simulink model "P2_SIL_Model_Diag"  (R2016a)
settings: Solver=ode2  StartTime=0.0  StopTime=Cycle_End  RelTol=1e-3
undefined symbols (not defined in the file): air, APP1_OOR, APP2_OOR, APP_Conversion_IN, APP_Mismatch, bms_inletair_temp, bms_maxchargecurrent, bms_maxdischargecurrent, BMS_Notfallkuehlung, BPP_Flt, cal, clt, ClutchEngag, CrankRequest, dcdc, eng, Engine, EngOverTemp, ENGTRQ_MSMCH_Degraded_CP, ENGTRQ_MSMCH_ErrCritical_CP, ENGTRQ_MSMCH_LimpHome_CP, EngTrqMismatch, env, ess, ESS, ESSOverTemp, fd, FFD, g, gb, Grade, IMG, KeyPos_Flt, KeyPosition, lib_APP_Conversion_IN, lib_ESS_plant_V1_2, lib_OBC_Manager, LossCAN, max_vehicle_rad_air_flow, MCUOverTemp, mot, MotDirMismatch, MotOverTemp, MotTrqMismatch, mph2kph, mph2ms, NeutralGear, obc, OBC_Manager, ParkGear, PRNDL_Flt, ReverseGear, RFD, rho, ShiftLeverPosition, sigbuilder_block, Speed, t_amb, time, tloop ... (+2)
libraries: simulink x104, EC2_libraries x12, Diagnostic x11, lib_CANerror_Detect x3, Utility x1
(part 2 of 11)

== system P2_SIL_Model_Diag/Camaro Plant Model/ESS/ESS ==
  note: Sensors
  note: Discharge is Negative!
  note: $Author: eo1000 $
      | $Rev: 431 $
      | $Date: 2016-09-24 14:28:33 -0500 (Sat, 24 Sep 2016) $
  "In " : Inport
  "Crr " : Inport  Port=2
  0 current : Memory  InheritSampleTime=on
  Bus Creator1 : BusCreator  Inputs=5
  Constant{1..4} (4 alike) : Constant  Value=0
  Data Type Conversion : DataTypeConversion  OutDataTypeStr=double
  ESSThermal : Subsystem
  Gain : Gain  Gain=3
  LoadCharacteristics : Subsystem
  Switch : Switch  Threshold=1
  Switch1 : Switch  Threshold=1
  Switch2 : Switch  Threshold=1
  Switch3 : Switch  Threshold=5
  Switch4 : Switch  Threshold=5
  To Workspace4 : ToWorkspace  VariableName=ess_current_hist  SampleTime=-1
      settings: Decimation=WORKSPACE_DECIMATION
  To Workspace5 : ToWorkspace  VariableName=ess_term_voltage_hist  SampleTime=-1
      settings: Decimation=WORKSPACE_DECIMATION
  To Workspace6 : ToWorkspace  VariableName=ess_mainc_hist  SampleTime=-1
      settings: Decimation=WORKSPACE_DECIMATION
  output voltage limits : Saturate  UpperLimit=ess.plant.init.series_cells*ess.plant.init.cell_max_V  LowerLimit=ess.plant.init.series_cells*ess.plant.init.cell_min_V
  tloop1 : Gain  Gain=-1
  tloop2 : Gain  Gain=1/ess.plant.init.series_cells
  out : Outport
  Voltage : Outport  Port=2
  wires:
  "In "/1 -> [ess_mainc_stat]
  Bus Creator1/1 -> out/1
  Data Type Conversion/1 -> To Workspace6/1
  LoadCharacteristics/1(Vterm) -> output voltage limits/1  "v_term"
  LoadCharacteristics/2(Resistance) -> ESSThermal/1(Resistance)
  tloop1/1 -> 0 current/1
  Constant2/1 -> Switch1/3
  Switch1/1 -> To Workspace4/1  "ess_ibat"
  output voltage limits/1 -> Switch2/1, tloop2/1  "output voltage"
  [ess_mainc_stat] -> Switch3/2, Data Type Conversion/1, Switch3/3  "MainC"
  Constant3/1 -> Switch2/3
  Switch2/1 -> To Workspace5/1, Voltage/1, Bus Creator1/1  "ess_vbat"
  [SOC] -> Bus Creator1/5  "ess_soc"
  tloop2/1 -> Bus Creator1/3  "Vcell"
  Constant1/1 -> Switch3/1
  Switch3/1 -> Switch1/2
  [ess_mainc_stat] -> Switch4/3, Switch4/2  "MainC"
  Constant4/1 -> Switch4/1
  Switch4/1 -> Switch2/2
  0 current/1 -> LoadCharacteristics/1(Current), ESSThermal/2(Current), Bus Creator1/4, Switch1/1  "ess_ibat"
  "Crr "/1 -> tloop1/1  "current"
  [ESSOverTemp] -> Switch/2
  Switch/1 -> Bus Creator1/2  "temp"
  ESSThermal/1(Temp[degC]) -> Switch/3, Gain/1  "temp"
  Gain/1 -> Switch/1

== system P2_SIL_Model_Diag/Camaro Plant Model/ESS/Inputs ==
  Bus Creator1 : BusCreator  Inputs=2
  CAN_fromHCU : Subsystem
  Digital_fromHCU : Subsystem
  Inputs : Outport
  wires:
  Digital_fromHCU/1(Outputs) -> Bus Creator1/2  "Digital"
  CAN_fromHCU/1(Outputs) -> Bus Creator1/1  "CAN"
  Bus Creator1/1 -> Inputs/1

== system P2_SIL_Model_Diag/Camaro Plant Model/ESS/Outputs ==
  Outputs : Inport
  tag scope: BMS_to_HCU=global
  wires:
  Outputs/1 -> [BMS_to_HCU]  "BMS_CAN"

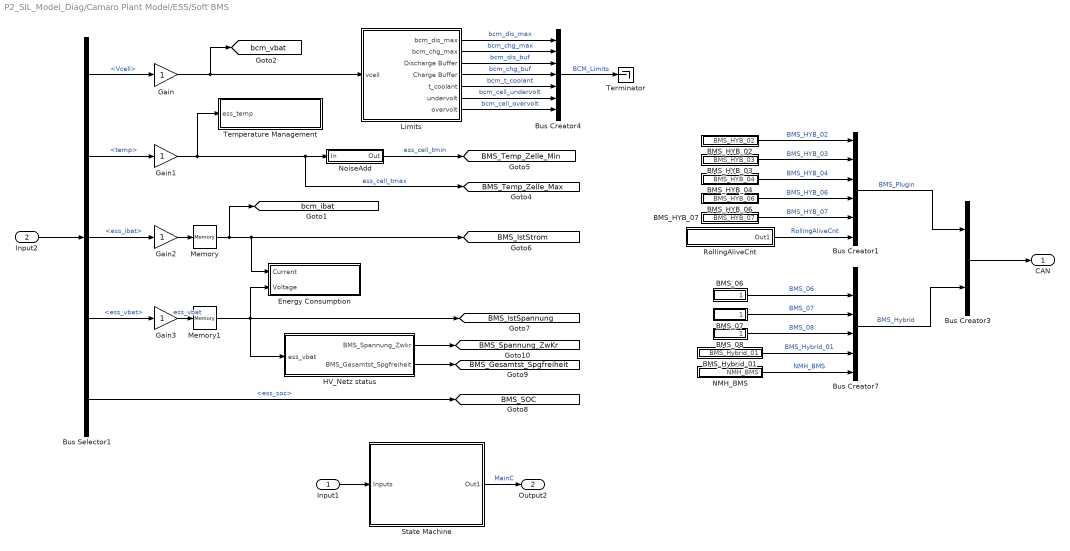
== system P2_SIL_Model_Diag/Camaro Plant Model/ESS/Soft BMS ==
  Input1 : Inport
  Input2 : Inport  Port=2
  BMS_06 : Subsystem
  BMS_07 : Subsystem
  "BMS_08 " : Subsystem
  BMS_HYB_02 : Subsystem
  BMS_HYB_03 : Subsystem
  BMS_HYB_04 : Subsystem
  BMS_HYB_06 : Subsystem
  BMS_HYB_07 : Subsystem
  BMS_Hybrid_01 : Subsystem
  Bus Creator1 : BusCreator  Inputs=6
  Bus Creator3 : BusCreator  Inputs=2
  Bus Creator4 : BusCreator  Inputs=7
  Bus Creator7 : BusCreator  Inputs=6
  Bus Selector1 : BusSelector  OutputSignals=Vcell,temp,ess_ibat,ess_vbat,ess_soc
  Energy Consumption : Subsystem
  Gain{,1..3} (4 alike) : Gain
  HV_Netz status : Subsystem
  Limits : Subsystem
  Memory : Memory
  Memory1 : Memory
  NMH_BMS : Subsystem
  NoiseAdd : Subsystem
  RollingAliveCnt : Subsystem
  State Machine : Subsystem
  Temperature Management : Subsystem
  Terminator : Terminator
  CAN : Outport
  Output2 : Outport  Port=2
  tag scope: BMS_Gesamtst_Spgfreiheit=global, BMS_IstSpannung=global, BMS_IstStrom=global, BMS_SOC=global, BMS_Spannung_ZwKr=global, BMS_Temp_Zelle_Max=global, BMS_Temp_Zelle_Min=global, bcm_ibat=global, bcm_vbat=global
  wires:
  State Machine/1(Out1) -> Output2/1  "MainC"
  Gain3/1 -> Memory1/1  "ess_vbat"
  Gain2/1 -> Memory/1
  Gain/1 -> [bcm_vbat], Limits/1(vcell)
  Input1/1 -> State Machine/1(Inputs)
  Input2/1 -> Bus Selector1/1
  Bus Selector1/3 -> Gain2/1  "<ess_ibat>"
  Bus Creator1/1 -> Bus Creator3/1  "BMS_Plugin"
  NoiseAdd/1(Out) -> [BMS_Temp_Zelle_Min]  "ess_cell_tmin"
  Bus Selector1/1 -> Gain/1  "<Vcell>"
  Bus Selector1/2 -> Gain1/1  "<temp>"
  Gain1/1 -> Temperature Management/1(ess_temp), NoiseAdd/1(In), [BMS_Temp_Zelle_Max]  "ess_cell_tmax"
  Limits/1(bcm_dis_max) -> Bus Creator4/1  "bcm_dis_max"
  Limits/3(Discharge Buffer) -> Bus Creator4/3  "bcm_dis_buf"
  Limits/4(Charge Buffer) -> Bus Creator4/4  "bcm_chg_buf"
  Limits/5(t_coolant) -> Bus Creator4/5  "bcm_t_coolant"
  Limits/2(bcm_chg_max) -> Bus Creator4/2  "bcm_chg_max"
  Bus Creator4/1 -> Terminator/1  "BCM_Limits"
  Bus Selector1/5 -> [BMS_SOC]  "<ess_soc>"
  Bus Selector1/4 -> Gain3/1  "<ess_vbat>"
  Limits/6(undervolt) -> Bus Creator4/6  "bcm_cell_undervolt"
  Limits/7(overvolt) -> Bus Creator4/7  "bcm_cell_overvolt"
  Bus Creator7/1 -> Bus Creator3/2  "BMS_Hybrid"
  "BMS_08 "/1(BMS_08) -> Bus Creator7/4  "BMS_08"
  BMS_06/1(BMS_06) -> Bus Creator7/2  "BMS_06"
  BMS_HYB_06/1(BMS_HYB_06) -> Bus Creator1/4  "BMS_HYB_06"
  BMS_HYB_02/1(BMS_HYB_02) -> Bus Creator1/1  "BMS_HYB_02"
  BMS_HYB_04/1(BMS_HYB_04) -> Bus Creator1/3  "BMS_HYB_04"
  BMS_07/1(BMS_07) -> Bus Creator7/3  "BMS_07"
  BMS_Hybrid_01/1(BMS_Hybrid_01) -> Bus Creator7/5  "BMS_Hybrid_01"
  BMS_HYB_07/1(BMS_HYB_07) -> Bus Creator1/5  "BMS_HYB_07"
  BMS_HYB_03/1(BMS_HYB_03) -> Bus Creator1/2  "BMS_HYB_03"
  NMH_BMS/1(NMH_BMS) -> Bus Creator7/6  "NMH_BMS"
  Bus Creator3/1 -> CAN/1
  HV_Netz status/1(BMS_Spannung_Zwkr) -> [BMS_Spannung_ZwKr]
  HV_Netz status/2(BMS_Gesamtst_Spgfreiheit) -> [BMS_Gesamtst_Spgfreiheit]
  Memory/1 -> [bcm_ibat], Energy Consumption/1(Current), [BMS_IstStrom]
  Memory1/1 -> [BMS_IstSpannung], HV_Netz status/1(ess_vbat), Energy Consumption/2(Voltage)
  RollingAliveCnt/1(Out1) -> Bus Creator1/6  "RollingAliveCnt"

== system P2_SIL_Model_Diag/Camaro Plant Model/ICE Simple1/Engine Plant Modified ==
  "In " : Inport
  eng_spd_out : Inport  Port=2
  Core Engine : Subsystem
      mask Display: image(imread('EngineShortBlock.jpg'),'center')
  ECU Actuators : Subsystem
  ECU Sensors : Subsystem
  Fuel Supply : Subsystem
      mask Display: image(imread('FuelTank.jpg'),'center')
  Radiator : Subsystem  Commented=on  AncestorBlock=lib_Vehicle/Vehicle_Plant_Model/Radiator
  Out : Outport
  eng_shaft_out : Outport  Port=2
  tag scope: EngCrankCmd=global, EngRunAtv=global, EngShutdown=global, Eng_Fan=global, Eng_Temp=global, FuelPumpEnable=global, ThrPstCmd_pct=global, VehSpdAvgDrvn_Eng=global
  wires:
  ECU Actuators/5(Out5) -> [EngShutdown]
  [FuelLevelPct] -> ECU Sensors/4(In4)  "FuelLevelPct"
  [EmsHC] -> ECU Sensors/6(In6)  "HC_g/s"
  [EngPe] -> ECU Sensors/5(In5)  "PE_0_1"
  [EmsCO] -> ECU Sensors/7(In7)  "CO_g/s"
  [EmsCO2] -> ECU Sensors/8(In8)  "CO2_g/s"
  [EmsNOx] -> ECU Sensors/9(In9)  "NOx_g/s"
  Fuel Supply/1(Available Fuel) -> Core Engine/2(Available Fuel)
  ECU Actuators/4(Out4) -> [FuelPumpEnable]
  ECU Actuators/1(Out1) -> [ThrPstCmd_pct]
  "In "/1 -> ECU Actuators/1(In1)
  [EngBrkTrq] -> ECU Sensors/1(In1)  "EngActStdyStTorq_Nm"
  [AdvFuelFlowEst] -> ECU Sensors/3(In3)  "EngFuelFlow_g/s"
  [EngSpd_RPM] -> ECU Sensors/2(In2)  "EngSpd_RPM"
  ECU Actuators/2(Out2) -> [EngCrankCmd]
  ECU Actuators/3(Out3) -> [EngRunAtv]
  Core Engine/1(eng_shaft_out) -> eng_shaft_out/1
  eng_spd_out/1 -> Core Engine/1(Engine Speed (rad/s))
  [EngTemp] -> ECU Sensors/10(In10)  "Eng_Temp"
  [Eng_Fan] -> Radiator/2(Fans)
  [Eng_Temp] -> Radiator/1(EngCltTmp)
  ECU Actuators/6(Out6) -> [Eng_Temp]
  ECU Actuators/7(Out7) -> [Eng_Fan]
  ECU Actuators/8(Out8) -> [VehSpdAvgDrvn_Eng]
  ECU Sensors/1(Out1) -> Out/1

== system P2_SIL_Model_Diag/Camaro Plant Model/ICE Simple1/Inputs ==
  Analog : Subsystem
  Bus Creator : BusCreator  Inputs=2
  CAN_from_HCU : Subsystem
  Inputs : Outport
  wires:
  CAN_from_HCU/1(Out1) -> Bus Creator/1  "CAN"
  Analog/1(Out1) -> Bus Creator/2  "Analog"
  Bus Creator/1 -> Inputs/1

== system P2_SIL_Model_Diag/Camaro Plant Model/ICE Simple1/Soft ECM ==
  note: Should check lookup table with GM
  In : Inport
  In1 : Inport  Port=2
  Bus Creator1 : BusCreator  Inputs=3
  Bus Creator2 : BusCreator  Inputs=10
  Bus Selector : BusSelector  OutputSignals=EngSpd_RPM
  Bus Selector1 : BusSelector  OutputSignals=CAN.to EBCAN.ECM_CAN.EngTrqCmd,CAN.to EBCAN.ECM_CAN.EngAppReq,CAN.to VEH_CAN.to_BCM.SysPwrMd,CAN.to EBCAN.ECM_CAN.ShftLvrPos
  Bus Selector2 : BusSelector  OutputSignals=Eng_Temp,EngFuelFlow_g/s
  Data Type Conversion4 : DataTypeConversion
  ECM_RollingAliveCnt : Subsystem
  Fuel Consumption : Subsystem
  Logic : Stateflow chart  TreatAsAtomicUnit=on
  Memory1 : Memory  X0=Engine.Init_T_amb
  Memory2 : Memory
  temp vs fan : Lookup_n-D  NumberOfTableDimensions=1  BreakpointsForDimension1=[0:1:100]  Table=[0:0.01:1]  InternalRulePriority=Speed  RndMeth=Simplest  InputSameDT=on
  Out : Outport
  Out1 : Outport  Port=2
  wires:
  Logic/3(EngRunAtv) -> Bus Creator2/4  "EngRunAtv"
  Bus Selector/1 -> Logic/4(EngSpd_RPM)  "<EngSpd_RPM>"
  Bus Selector1/2 -> Memory2/1  "<EngAppReq>"
  Logic/2(EngCrankCmd) -> Bus Creator2/3  "Eng12vStrtrMtrCmmdOn"
  Bus Creator1/1 -> Out/1  "ECM_CAN"
  Bus Creator2/1 -> Out1/1, Bus Creator1/1  "ECM_to_Actuators"
  Logic/1(ThrottleCmd) -> Bus Creator2/2  "ThrPosCmd_%"
  In1/1 -> Bus Selector2/1, Bus Creator1/3, Bus Selector/1  "Sensors_to_ECM"
  In/1 -> Bus Selector1/1  "HCU_to_ECM"
  Logic/4(FuelPumpEnable) -> Bus Creator2/5  "FuelPumpEnable"
  Bus Selector1/3 -> Logic/2(SysPwrMd)  "<SysPwrMd>"
  [VehSpdAvgDrvn] -> Bus Creator2/7, Logic/5(VehSpdAvgDrvn)  "VehSpdAvgDrvn"
  Bus Selector1/4 -> Logic/3(ShftLvrPos)  "<ShftLvrPos>"
  Logic/5(EngShutdown) -> Bus Creator2/6  "EngShutdown"
  Bus Selector2/1 -> Memory1/1, temp vs fan/1  "<Eng_Temp>"
  Bus Selector2/2 -> Fuel Consumption/1(Fuel Consumption)  "<EngFuelFlow_g/s>"
  Fuel Consumption/1(fuel consumption) -> Bus Creator1/2  "Eng_fuel_consumption"
  temp vs fan/1 -> Bus Creator2/10  "fan_cmd"
  Memory1/1 -> Bus Creator2/9  "Eng_Temp"
  Memory2/1 -> Logic/1(drvAPP)
  Bus Selector1/1 -> Data Type Conversion4/1  "<EngTrqCmd>"
  Data Type Conversion4/1 -> Bus Creator2/1  "EngTrqCmd"
  ECM_RollingAliveCnt/1(Out1) -> Bus Creator2/8

== system P2_SIL_Model_Diag/Camaro Plant Model/IMG/IMG Plant ==
  "In1 " : Inport
  voltage : Inport  Port=2
  MotShaftIn : Inport  Port=3
  SpdOut : Inport  Port=4
  " Actuators" : Subsystem
  Clutch : Subsystem
      mask Display:
      | image('Images\Clutch.png')
      | color('red');
      | port_label('Input',1,'Cmd')
      | port_label('Input',2,'ShaftIn')
      | port_label('Input',3,'SpdOut')
      | port_label('Output',1,'ShaftOut')
      | port_label('Output',2,'SpdIn')
  Electric Machine : Subsystem
      mask Display:
      | image('Images\Motor.png')
      | color('red');
      | port_label('Input',1,'MotTrqCmd');
      | port_label('Input',2,'Volt');
      | port_label('Input',3,'ShaftIn');
      | port_label('Input',4,'SpdOut');
      | port_label('Output',1,'Crr')
      | port_label('Output',2,'SpdIn')
  Sensors : Subsystem
  Out1 : Outport
  current : Outport  Port=2
  MotShaftOut : Outport  Port=3
  SpdIn : Outport  Port=4
  wires:
  [LockupCmd] -> Clutch/1(clt_lockup_cmd)
  [mot_temp] -> Sensors/5(In6)
  [mot_spd_out] -> Sensors/1(In2)
  [mot_crr_out] -> Sensors/3(In4)
  "In1 "/1 -> " Actuators"/1(In1)
  [mot_volt_in] -> Sensors/4(In5)
  " Actuators"/1(Out2) -> [MotTrqCmd]
  Sensors/1(Out1) -> Out1/1
  [mot_trq_out] -> Sensors/2(In3)
  Clutch/2(ctl_spd_in) -> SpdIn/1
  SpdOut/1 -> Electric Machine/4(MotSpdOut)
  Clutch/1(clt_shaft_out) -> Electric Machine/3(mot_trq_in mot_inertia_in)
  Electric Machine/2(mot_trq_out mot_inertia_out) -> MotShaftOut/1
  MotShaftIn/1 -> Clutch/2(clt_trq_in clt_inertia_in)
  Electric Machine/3(MotSpdIn) -> Clutch/3(clt_spd_out)
  Electric Machine/1(mot_current_out) -> current/1
  [MotTrqCmd] -> Electric Machine/1(MotTrqCmd)
  " Actuators"/2(Out1) -> [LockupCmd]
  voltage/1 -> Electric Machine/2(voltage)
  [mcu_temp] -> Sensors/6(In1)
  [clt_plant_spd_in] -> Sensors/7(In7)

== system P2_SIL_Model_Diag/Camaro Plant Model/IMG/Soft MCU ==
  In : Inport
  In1 : Inport  Port=2
  Bus Creator : BusCreator  Inputs=6
  Bus Creator1 : BusCreator  Inputs=2
  Bus Selector : BusSelector  OutputSignals=mot_spd_out,mot_trq_out
  Bus Selector1 : BusSelector  OutputSignals=to_MCU.ClutchEngage,to_MCU.Inverter_Enable,to_MCU.Torque_Command
  Constant : Constant  Value=0
  Data Type Conversion{,1..4} (5 alike) : DataTypeConversion
  MCU_CAN_rolling : Subsystem
  Memory : Memory
  Switch : Switch  Threshold=1
  Torque Calculation : Subsystem
  Out : Outport
  Out1 : Outport  Port=2
  wires:
  In1/1 -> Bus Creator1/2, Bus Selector/1  "Sensors_to_MCU"
  Bus Creator1/1 -> Out/1  "MCU_CAN"
  In/1 -> Bus Selector1/1  "HCU_to_MCU"
  Bus Selector1/3 -> Data Type Conversion4/1, Torque Calculation/1(MotTrqReq)  "<Torque_Command>"
  Bus Creator/1 -> Bus Creator1/1, Out1/1  "MCU_to _Actuator"
  Bus Selector1/2 -> Memory/1, Switch/2  "<Inverter_Enable>"
  Constant/1 -> Switch/3
  Bus Selector1/1 -> Data Type Conversion/1  "<ClutchEngage>"
  Data Type Conversion/1 -> Bus Creator/2  "EngageClutch"
  Bus Selector/1 -> Torque Calculation/2(MotSpd)  "<mot_spd_out>"
  Torque Calculation/1(mot_trq_out) -> Switch/1
  Data Type Conversion1/1 -> Bus Creator/4  "InverterEnabled"
  Bus Selector/2 -> Torque Calculation/3(MotTrqFdbck), Data Type Conversion2/1  "<mot_trq_out>"
  Data Type Conversion2/1 -> Bus Creator/5  "MotTrqFdbck"
  Memory/1 -> Data Type Conversion1/1
  Switch/1 -> Data Type Conversion3/1  "MotTrqCmd"
  Data Type Conversion3/1 -> Bus Creator/3  "MotTrqCmd"
  Data Type Conversion4/1 -> Bus Creator/1  "Torque_Command"
  MCU_CAN_rolling/1(Out1) -> Bus Creator/6  "RollingAliveCnt"

== system P2_SIL_Model_Diag/Camaro Plant Model/On-Board Charger/HCU to OBC ==
  Bus Creator1 : BusCreator  Inputs=2
  CAN_fromHCU : Subsystem
  Digital_fromHCU : Subsystem
  Inputs : Outport
  wires:
  Digital_fromHCU/1(Outputs) -> Bus Creator1/2
  CAN_fromHCU/1(Outputs) -> Bus Creator1/1
  Bus Creator1/1 -> Inputs/1

== system P2_SIL_Model_Diag/Camaro Plant Model/On-Board Charger/OBC to HCU ==
  Outputs : Inport
  Bus Selector : BusSelector  OutputSignals=OBC_CAN
  tag scope: OBC_to_HCU=global
  wires:
  Bus Selector/1 -> [OBC_to_HCU]  "<OBC_CAN>"
  Outputs/1 -> Bus Selector/1

== system P2_SIL_Model_Diag/Camaro Plant Model/On-Board Charger/On Board Charger ==
  "In1 " : Inport
  volt : Inport  Port=2
  " Actuators" : Subsystem
  Bus Selector : BusSelector  OutputSignals=EVSE_Plugged
  Constant : Constant  Value=obc.plant.init.Level1ChargerVoltage
  Constant1 : Constant  Value=obc.plant.init.Level2ChargerVoltage
  Constant{2,4..7} (5 alike) : Constant  Value=0
  Constant3 : Constant  Value=obc.plant.init.OutputPower
  Index Vector : MultiPortSwitch  DataPortOrder=Zero-based contiguous  zeroidx=on
  Sensors : Subsystem
  Subsystem2 : Subsystem
      mask Display: disp('divider')
  Terminator : Terminator
  "charging current polarity " : Gain  Gain=-1
  Out1 : Outport
  crr : Outport  Port=2
  wires:
  "charging current polarity "/1 -> crr/1
  Constant3/1 -> Subsystem2/1(In1)
  volt/1 -> Terminator/1
  Subsystem2/1(Out1) -> "charging current polarity "/1
  Constant2/1 -> Index Vector/2
  Constant/1 -> Index Vector/3
  Constant1/1 -> Index Vector/4
  [Driver_Request] -> Bus Selector/1
  Bus Selector/1 -> Index Vector/1  "<EVSE_Plugged>"
  Index Vector/1 -> Subsystem2/2(In2)
  Constant4/1 -> Sensors/1(In2)
  Constant6/1 -> Sensors/3(In4)
  Constant7/1 -> Sensors/4(In5)
  Sensors/1(Out1) -> Out1/1
  Constant5/1 -> Sensors/2(In3)
  "In1 "/1 -> " Actuators"/1(In1)
  " Actuators"/1(Out2) -> [Enable]
  " Actuators"/2(Out1) -> [NLG5_MC_MAX]
  " Actuators"/3(Out3) -> [NLG5_OC_COM]
  " Actuators"/4(Out4) -> [VoltageEnable]

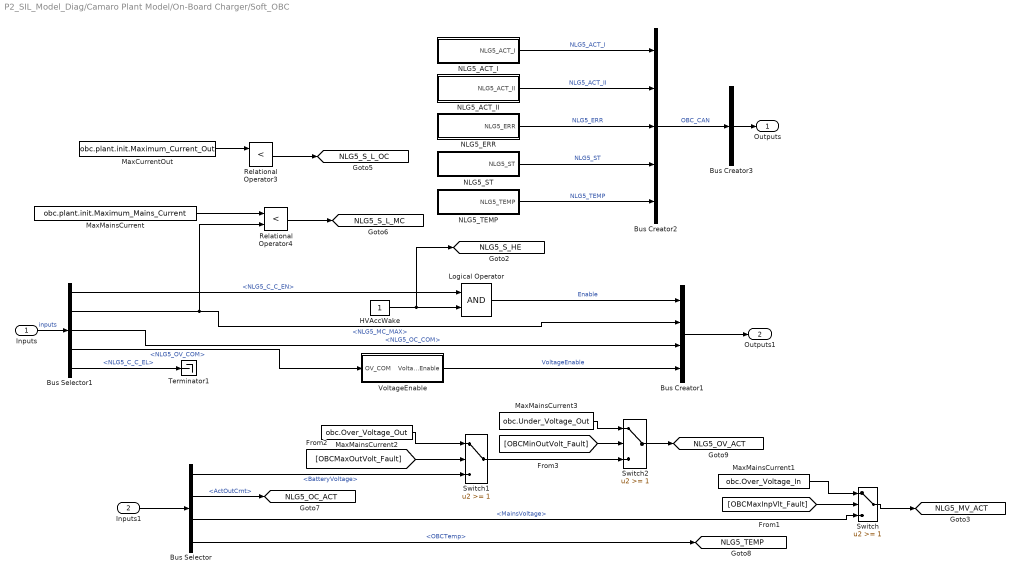
== system P2_SIL_Model_Diag/Camaro Plant Model/On-Board Charger/Soft_OBC ==
  Inputs : Inport
  Inputs1 : Inport  Port=2
  Bus Creator1 : BusCreator  Inputs=4
  Bus Creator2 : BusCreator  Inputs=5
  Bus Creator3 : BusCreator  Inputs=1
  Bus Selector : BusSelector  OutputSignals=BatteryVoltage,ActOutCrnt,MainsVoltage,OBCTemp
  Bus Selector1 : BusSelector  OutputSignals=to HV_CAN.to_OBC.NLG5_C_C_EN,to HV_CAN.to_OBC.NLG5_MC_MAX,to HV_CAN.to_OBC.NLG5_OC_COM,to HV_CAN.to_OBC.NLG5_OV_COM,to HV_CAN.to_OBC.NLG5_C_C_EL
  HVAccWake : Constant
  Logical Operator : Logic  AllPortsSameDT=off  OutDataTypeStr=boolean
  MaxCurrentOut : Constant  Value=obc.plant.init.Maximum_Current_Out
  MaxMainsCurrent : Constant  Value=obc.plant.init.Maximum_Mains_Current
  MaxMainsCurrent1 : Constant  Value=obc.Over_Voltage_In
  MaxMainsCurrent2 : Constant  Value=obc.Over_Voltage_Out
  MaxMainsCurrent3 : Constant  Value=obc.Under_Voltage_Out
  NLG5_ACT_I : Subsystem
  NLG5_ACT_II : Subsystem
  NLG5_ERR : Subsystem
  NLG5_ST : Subsystem
  NLG5_TEMP : Subsystem
  Relational Operator3 : RelationalOperator  Operator=<  OutDataTypeStr=boolean
  Relational Operator4 : RelationalOperator  Operator=<  OutDataTypeStr=boolean
  Switch : Switch  Threshold=1
  Switch1 : Switch  Threshold=1
  Switch2 : Switch  Threshold=1
  Terminator1 : Terminator
  VoltageEnable : Subsystem
  Outputs : Outport
  Outputs1 : Outport  Port=2
  tag scope: NLG5_MV_ACT=global, NLG5_OC_ACT=global, NLG5_OV_ACT=global, NLG5_S_HE=global, NLG5_S_L_MC=global, NLG5_S_L_OC=global, NLG5_TEMP=global
  wires:
  NLG5_ST/1(NLG5_ST) -> Bus Creator2/4  "NLG5_ST"
  VoltageEnable/1(VoltageEnable) -> Bus Creator1/4  "VoltageEnable"
  Bus Selector1/5 -> Terminator1/1  "<NLG5_C_C_EL>"
  Bus Selector1/1 -> Logical Operator/1  "<NLG5_C_C_EN>"
  Inputs/1 -> Bus Selector1/1  "inputs"
  NLG5_TEMP/1(NLG5_TEMP) -> Bus Creator2/5  "NLG5_TEMP"
  NLG5_ERR/1(NLG5_ERR) -> Bus Creator2/3  "NLG5_ERR"
  NLG5_ACT_II/1(NLG5_ACT_II) -> Bus Creator2/2  "NLG5_ACT_II"
  Bus Creator3/1 -> Outputs/1
  Bus Creator2/1 -> Bus Creator3/1  "OBC_CAN"
  NLG5_ACT_I/1(NLG5_ACT_I) -> Bus Creator2/1  "NLG5_ACT_I"
  Inputs1/1 -> Bus Selector/1
  Bus Creator1/1 -> Outputs1/1
  Logical Operator/1 -> Bus Creator1/1  "Enable"
  MaxCurrentOut/1 -> Relational Operator3/1
  Relational Operator3/1 -> [NLG5_S_L_OC]
  MaxMainsCurrent/1 -> Relational Operator4/1
  Relational Operator4/1 -> [NLG5_S_L_MC]
  Bus Selector/2 -> [NLG5_OC_ACT]  "<ActOutCrnt>"
  [OBCMaxInpVlt_Fault] -> Switch/2
  Bus Selector/3 -> Switch/3  "<MainsVoltage>"
  MaxMainsCurrent1/1 -> Switch/1
  Switch/1 -> [NLG5_MV_ACT]
  [OBCMaxOutVolt_Fault] -> Switch1/2
  MaxMainsCurrent2/1 -> Switch1/1
  Bus Selector/1 -> Switch1/3  "<BatteryVoltage>"
  Bus Selector/4 -> [NLG5_TEMP]  "<OBCTemp>"
  Switch1/1 -> Switch2/3
  Switch2/1 -> [NLG5_OV_ACT]
  [OBCMinOutVolt_Fault] -> Switch2/2
  MaxMainsCurrent3/1 -> Switch2/1
  HVAccWake/1 -> [NLG5_S_HE], Logical Operator/2
  Bus Selector1/2 -> Relational Operator4/2, Bus Creator1/2  "<NLG5_MC_MAX>"
  Bus Selector1/3 -> Bus Creator1/3  "<NLG5_OC_COM>"
  Bus Selector1/4 -> VoltageEnable/1(OV_COM)  "<NLG5_OV_COM>"

== system P2_SIL_Model_Diag/Camaro Plant Model/Transmission1/Inputs ==
  Analog_fromHCU : Subsystem
  Bus Creator1 : BusCreator  Inputs=3
  CAN_fromHCU : Subsystem
  Digital_fromHCU : Subsystem
  Inputs : Outport
  wires:
  Digital_fromHCU/1(Outputs) -> Bus Creator1/2  "Digital"
  CAN_fromHCU/1(Outputs) -> Bus Creator1/1  "CAN"
  Bus Creator1/1 -> Inputs/1
  Analog_fromHCU/1(Outputs) -> Bus Creator1/3

== system P2_SIL_Model_Diag/Camaro Plant Model/Transmission1/Outputs ==
  Outputs : Inport
  tag scope: TCM_to_HCU=global
  wires:
  Outputs/1 -> [TCM_to_HCU]  "TCM_CAN"

== system P2_SIL_Model_Diag/Camaro Plant Model/Transmission1/Soft TCM ==
  In : Inport
  In1 : Inport  Port=2
  6L45 Logic : Stateflow chart  TreatAsAtomicUnit=on
  Bus Creator : BusCreator  Inputs=3
  Bus Creator1 : BusCreator  Inputs=2
  Bus Selector : BusSelector  OutputSignals=impeller_spd_rads,turbine_spd_rads
  Bus Selector1 : BusSelector  OutputSignals=CAN.to_TCM.AccPos_Perc,CAN.to_TCM.VehSpdAvgDrvn_kph
  Constant : Constant  Value=4
  Conversion  APP1 (%) : DataTypeConversion  OutDataTypeStr=int8
  Sum : Sum  Inputs=|++
  Switch : Switch  Threshold=1
  TorqConv Lockup threshold : Constant  Value=tc.plant.init.lock_thresh
  Out : Outport
  Out1 : Outport  Port=2
  wires:
  TorqConv Lockup threshold/1 -> 6L45 Logic/1(tc_lockup_thrsh)
  6L45 Logic/1(TransEstGear) -> Bus Creator/1
  [ShftLvrPos] -> Switch/3, Sum/1  "TrnsShftLvrPos"
  In1/1 -> Bus Selector/1, Bus Creator1/2  "Sensors_to_TCM"
  Bus Creator1/1 -> Out/1  "TCM_CAN"
  In/1 -> Bus Selector1/1  "HCU_to_TCM"
  Bus Selector/2 -> 6L45 Logic/5(tc_spd_out)  "<turbine_spd_rads>"
  Bus Selector/1 -> 6L45 Logic/4(tc_spd_in)  "<impeller_spd_rads>"
  Bus Selector1/2 -> 6L45 Logic/3(VehicleSpeed)  "<VehSpdAvgDrvn_kph>"
  Bus Selector1/1 -> 6L45 Logic/2(drvAPP)  "<AccPos_Perc>"
  Bus Creator/1 -> Out1/1, Bus Creator1/1  "TCM_to _Actuator"
  6L45 Logic/2(LockupCmd) -> Bus Creator/2
  [drv_BPP_percent] -> 6L45 Logic/6(drvBPP)
  Sum/1 -> Switch/1
  [PRNDL_Flt_ON] -> Switch/2
  Switch/1 -> 6L45 Logic/7(ShftLvrPos), Bus Creator/3  "TrnsShftLvrPos"
  Constant/1 -> Conversion  APP1 (%)/1
  Conversion  APP1 (%)/1 -> Sum/2

== system P2_SIL_Model_Diag/Camaro Plant Model/Transmission1/Transmission Plant ==
  "In1 " : Inport
  TorqConvShaftIn : Inport  Port=2
  GearboxSpdOut : Inport  Port=3
  " Actuators" : Subsystem
  Gearbox : Subsystem
      mask Display:
      | image('Images\Gearbox.jpg')
      | color('red');
      | port_label('Input',1,'Gear');
      | port_label('Input',2,'ShftIn');
      | port_label('Input',3,'SpdOut');
      | port_label('Output',1,'ShaftOut');
      | port_label('Output',2,'SpdIn');
  Sensors : Subsystem
  Torque Converter : Subsystem
      mask Display:
      | image('Images\TorqConv.jpg')
      | color('red');
      | port_label('Input',2,'ShaftIn');
      | port_label('Input',3,'SpdOut');
      | port_label('Output',1,'ShaftOut');
      | port_label('Output',2,'SpdIn');
  Out1 : Outport
  GearboxShaftOut : Outport  Port=2
  TorqConvSpdIn : Outport  Port=3
  tag scope: TransEstGear=global
  wires:
  Torque Converter/2(cpl_spd_in) -> TorqConvSpdIn/1
  Gearbox/2(gb_spd_in) -> Torque Converter/3(tc_spd_out)
  TorqConvShaftIn/1 -> Torque Converter/2(tc_shaft_in)
  Gearbox/1(gb_trq_out gb_inertia_out) -> GearboxShaftOut/1
  " Actuators"/1(Out2) -> [TransEstGear]
  [tc_trq_out] -> Sensors/4(In5)
  [gb_spd_out] -> Sensors/5(In6)
  [gb_trq_out] -> Sensors/6(In7)
  [tc_spd_out] -> Sensors/2(In3)
  [tc_spd_in] -> Sensors/1(In2)
  [tc_trq_in] -> Sensors/3(In4)
  " Actuators"/2(Out5) -> [LockupCmd]
  "In1 "/1 -> " Actuators"/1(In1)
  Sensors/1(Out1) -> Out1/1
  [TransEstGear] -> Gearbox/1(TransEstGear)
  Torque Converter/1(tc_shaft_out) -> Gearbox/2(gb_trq_in gb_inertia_in)
  GearboxSpdOut/1 -> Gearbox/3(gb_spd_out)
  [LockupCmd] -> Torque Converter/1(tc_lockup)

== system P2_SIL_Model_Diag/Camaro Plant Model/Wheels/Force calculation ==
  spd in : Inport
  BPP[%] : Inport  Port=2
  whl_spd : Inport  Port=3
  grade : Inport  Port=4
  trq_in : Inport  Port=5
  "1\\radius " : Gain  Gain=1/whl.plant.init.radius  SaturateOnIntegerOverflow=on  OutDataTypeStr=Inherit: Same as input  ParamDataTypeStr=Inherit: Same as input
  1\radius 1 : Gain  Gain=-1/100  SaturateOnIntegerOverflow=on  OutDataTypeStr=Inherit: Same as input  ParamDataTypeStr=Inherit: Same as input
  Blending : Subsystem  mask(State dependent blending){xl=-0.1, yl=-1, xc=0, yc=0, xr=0.1, yr=1}
      mask prompts: xl "Left point (x-value):"; yl "Left point (y-value):"; xc "Center point (x-value):"; yc "Center point (y-value):"; xr "Right point (x-value):"; yr "Right point (y-vector):"
      mask Display: plot([-1 1 3 6 8], [1.5 1.5 0.5 4.0 4.0])
  Constant : Constant  Value=0
  Rolling Resistance : Subsystem
  Saturation1 : Saturate  UpperLimit=0  LowerLimit=-inf
  Sum2 : Sum  Inputs=++-  SaturateOnIntegerOverflow=on  InputSameDT=on  OutDataTypeStr=Inherit: Same as first input
  Switch : Switch  Threshold=1
  trq_brake_max : Gain  Gain=whl.plant.init.trq_brake_max
  force : Outport
  wires:
  Rolling Resistance/1(rolling resistence) -> Sum2/3
  grade/1 -> Rolling Resistance/2(grade)
  whl_spd/1 -> Rolling Resistance/1(whl_spd)
  Blending/1(Out1) -> Saturation1/1
  trq_brake_max/1 -> Blending/1(input)
  Sum2/1 -> "1\\radius "/1
  "1\\radius "/1 -> force/1
  Saturation1/1 -> Sum2/1
  BPP[%]/1 -> 1\radius 1/1  "brake cmd"
  spd in/1 -> Blending/2(Control (state))
  trq_in/1 -> Sum2/2
  [BPP_Flt] -> Switch/2
  Constant/1 -> Switch/1
  1\radius 1/1 -> Switch/3
  Switch/1 -> trq_brake_max/1

== system P2_SIL_Model_Diag/Camaro Plant Model/Wheels/Mass calculation ==
  inertia in : Inport
  1\radius^2 : Gain  Gain=1/whl.plant.init.radius^2  SaturateOnIntegerOverflow=on  OutDataTypeStr=Inherit: Same as input  ParamDataTypeStr=Inherit: Same as input
  Sum6 : Sum  SaturateOnIntegerOverflow=on  InputSameDT=on  OutDataTypeStr=Inherit: Same as first input
  wheel inertia : Constant  Value=whl.plant.init.inertia
  Mass : Outport
  wires:
  inertia in/1 -> Sum6/2
  1\radius^2/1 -> Mass/1
  Sum6/1 -> 1\radius^2/1
  wheel inertia/1 -> Sum6/1

== system P2_SIL_Model_Diag/Camaro Plant Model/Wheels/Speed calculation ==
  chas_spd : Inport
  spd in : Outport
  wires:
  chas_spd/1 -> spd in/1

== system P2_SIL_Model_Diag/Controller/HSC/Camaro Fault Detection ==
  Sensors : Inport
  Component Diagnostic : Subsystem
  Goto : Goto  Commented=on  GotoTag=ToDiagnostic
  Input Conversions : Subsystem
  Signal Diagnostic : Subsystem
  "Signal Generator " : Subsystem  Commented=on
  SystemDiag : Subsystem
  Out2 : Outport
  wires:
  Signal Diagnostic/1(Out2) -> Component Diagnostic/1(Sensors1)
  Component Diagnostic/1(Out2) -> SystemDiag/1(In1)
  "Signal Generator "/1(Out1) -> Goto/1
  Input Conversions/1(VehSig) -> Signal Diagnostic/1(VehSig)
  Sensors/1 -> Input Conversions/1(RawSig)
  SystemDiag/1(Out1) -> Out2/1

== system P2_SIL_Model_Diag/Controller/HSC/Driver_Requests ==
  Sensors : Inport
  Diagnostics : Inport  Port=2
  APP_BPP to DrvIntndAxlTrq1 : Subsystem  Commented=on  AncestorBlock=lib_APP_BPP_to_AxlTrq/APP_BPP to DrvIntndAxlTrq
  APP_BPP to DrvIntndAxlTrq2 : Subsystem  AncestorBlock=lib_APP_BPP_to_AxlTrq/APP_BPP to DrvIntndAxlTrq
  Vehicle_Shutdown : Subsystem  Commented=on  AncestorBlock=lib_Vehicle_Shutdown/Vehicle Shutdown
  Vehicle_Startup : Subsystem  RequirementInfo={'other' 'HCU_Requirements.xlsx' '@Simulink_requirement_item_7' 'true' 'Determines the vehicle readiness for driving and the vehicle readiness to enable the propulsion system' '' } %GIDa_f0db0623_b6ae_4f70_b976_36b3e85d9576  Commented=on  AncestorBlock=lib_Vehicle_Startup/Vehicle Startup
  DriverRequests : Outport
  wires:
  Sensors/1 -> Vehicle_Startup/1(Sensors), APP_BPP to DrvIntndAxlTrq2/1(Sensors), APP_BPP to DrvIntndAxlTrq1/1(Sensors), Vehicle_Shutdown/1(Sensors)
  APP_BPP to DrvIntndAxlTrq2/1(IntndAxlTrq) -> DriverRequests/1
  APP_BPP to DrvIntndAxlTrq1/1(IntndAxlTrq) -> ?  "DrvIntndAxlTrq"
  Vehicle_Shutdown/3(Components_Disabled) -> ?  "CmpnntsDsbld"
  Vehicle_Shutdown/2(HCUStatus) -> ?  "HCU_Status"
  APP_BPP to DrvIntndAxlTrq1/2(IntndAxlTrqStatus) -> ?  "IntndAxlTrqStatus"
  Diagnostics/1 -> Vehicle_Shutdown/2(Diagnostics)

== system P2_SIL_Model_Diag/Controller/HSC/Powertrain Manager ==
  Sensors : Inport
  Driver Request : Inport  Port=2
  Fault Detection : Inport  Port=3
  HV Manager : Subsystem
  Output Conversion : Subsystem
  PowertrainSUSD : Subsystem
  Torque Distribution : Subsystem  AncestorBlock=lib_Modes_manager/Modes Manager
  Out1 : Outport
  wires:
  [HV_BUS_Status] -> PowertrainSUSD/1(HV_Bus_Status)
  Sensors/1 -> Torque Distribution/1(Sensors), PowertrainSUSD/2(Sensors), HV Manager/1(Sensors)
  HV Manager/1(BMS_CAN) -> [BMS_CAN]
  HV Manager/2(HV_BUS_Status) -> [HV_BUS_Status]
  HV Manager/4(OBC_Status) -> [OBC_Status]
  PowertrainSUSD/1(MCU_CAN) -> [MCU_CAN]
  HV Manager/3(OBC_CAN) -> [OBC_CAN]
  PowertrainSUSD/2(MCU_Status) -> [MCU_Status]
  Torque Distribution/1(Controls) -> HV Manager/2(Controls), PowertrainSUSD/3(Control), [Controls]  "Controls"
  Driver Request/1 -> Torque Distribution/2(Driver Request)
  [BMS_CAN] -> Output Conversion/1(In1)  "BMS_CAN"
  [OBC_CAN] -> Output Conversion/2(In2)  "OBC_CAN"
  [MCU_CAN] -> Output Conversion/3(In3)  "MCU_CAN"
  [Controls] -> Output Conversion/4(In4)  "Controls"
  Output Conversion/1(Out1) -> Out1/1
  HV Manager/5(BMS_Digital) -> [BMS_Digital]
  [BMS_Digital] -> Output Conversion/5(In5)  "BMS_Digital"
  HV Manager/6(APM_CAN) -> [APM_CAN]
  HV Manager/7(APM_Status) -> [APM_Status]
  [APM_CAN] -> Output Conversion/6(In6)  "APM_CAN"
  Fault Detection/1 -> Torque Distribution/3(Fault Detection)

== system P2_SIL_Model_Diag/Fault Trigger Unit/Component Diagnostics setting/Mismch type ==
  In1 : Inport
  Constant : Constant  Value=cal.ENGTRQ_MSMCH.Degraded_CP+1
  Constant1 : Constant  Value=cal.ENGTRQ_MSMCH.LimpHome_CP+1
  Constant2 : Constant  Value=cal.ENGTRQ_MSMCH.ErrCritical_CP+1
  Constant3 : Constant  Value=0
  Multiport Switch : MultiPortSwitch  Inputs=4
  Out1 : Outport
  wires:
  Constant1/1 -> Multiport Switch/4
  Constant2/1 -> Multiport Switch/5
  In1/1 -> Multiport Switch/1
  Multiport Switch/1 -> Out1/1
  Constant3/1 -> Multiport Switch/2
  Constant/1 -> Multiport Switch/3

== system P2_SIL_Model_Diag/Fault Trigger Unit/Component Diagnostics setting/Mismch type1 ==
  In1 : Inport
  Constant : Constant  Value=cal.MOTTRQ_MSMCH.Degraded_CP+1
  Constant1 : Constant  Value=cal.MOTTRQ_MSMCH.LimpHome_CP+1
  Constant2 : Constant  Value=cal.ENGTRQ_MSMCH.ErrCritical_CP+1
  Constant3 : Constant  Value=0
  Multiport Switch : MultiPortSwitch  DataPortOrder=Zero-based contiguous  Inputs=4
  Out1 : Outport
  wires:
  Constant/1 -> Multiport Switch/3
  Constant3/1 -> Multiport Switch/2
  Multiport Switch/1 -> Out1/1
  In1/1 -> Multiport Switch/1
  Constant2/1 -> Multiport Switch/5
  Constant1/1 -> Multiport Switch/4

== system P2_SIL_Model_Diag/Fault Trigger Unit/Component Diagnostics setting/Override  ClutchEngag ==
  note: Override Switch Subsystem
  note: This subsystem is used to override the model value of a signal to a constant value
  In1 : Inport
  Constant : Constant  Value=0
  Multiport Switch : MultiPortSwitch  DataPortOrder=Zero-based contiguous  Inputs=2  zeroidx=on
  Signal Override Switch 0 = Use Model 1 = Use Constant : Constant  Value=0
  Out1 : Outport
  wires:
  Constant/1 -> Multiport Switch/3
  Multiport Switch/1 -> Out1/1
  In1/1 -> Multiport Switch/2
  Signal Override Switch 0 = Use Model 1 = Use Constant/1 -> Multiport Switch/1

== system P2_SIL_Model_Diag/Fault Trigger Unit/Component Diagnostics setting/Override  ESSOverTemp ==
  note: This subsystem is used to override the model value of a signal to a constant value
  note: Override Switch Subsystem
  In1 : Inport
  Constant : Constant  Value=0
  Multiport Switch : MultiPortSwitch  DataPortOrder=Zero-based contiguous  Inputs=2  zeroidx=on
  Signal Override Switch 0 = Use Model 1 = Use Constant : Constant  Value=0
  Out1 : Outport
  wires:
  Signal Override Switch 0 = Use Model 1 = Use Constant/1 -> Multiport Switch/1
  In1/1 -> Multiport Switch/2
  Multiport Switch/1 -> Out1/1
  Constant/1 -> Multiport Switch/3

== system P2_SIL_Model_Diag/Fault Trigger Unit/Component Diagnostics setting/Override  EngOverTemp ==
  note: Override Switch Subsystem
  note: This subsystem is used to override the model value of a signal to a constant value
  In1 : Inport
  Constant : Constant  Value=0
  Multiport Switch : MultiPortSwitch  DataPortOrder=Zero-based contiguous  Inputs=2  zeroidx=on
  Signal Override Switch 0 = Use Model 1 = Use Constant : Constant  Value=0
  Out1 : Outport
  wires:
  Constant/1 -> Multiport Switch/3
  Multiport Switch/1 -> Out1/1
  In1/1 -> Multiport Switch/2
  Signal Override Switch 0 = Use Model 1 = Use Constant/1 -> Multiport Switch/1

== system P2_SIL_Model_Diag/Fault Trigger Unit/Component Diagnostics setting/Override  EngTrqMismatch ==
  note: This subsystem is used to override the model value of a signal to a constant value
  note: Override Switch Subsystem
  In1 : Inport
  Constant : Constant  Value=0
  Multiport Switch : MultiPortSwitch  DataPortOrder=Zero-based contiguous  Inputs=2  zeroidx=on
  Signal Override Switch 0 = Use Model 1 = Use Constant : Constant  Value=0
  Out1 : Outport
  wires:
  Signal Override Switch 0 = Use Model 1 = Use Constant/1 -> Multiport Switch/1
  In1/1 -> Multiport Switch/2
  Multiport Switch/1 -> Out1/1
  Constant/1 -> Multiport Switch/3

== system P2_SIL_Model_Diag/Fault Trigger Unit/Component Diagnostics setting/Override  LossCAN ==
  note: Override Switch Subsystem
  note: This subsystem is used to override the model value of a signal to a constant value
  In1 : Inport
  Constant : Constant  Value=0
  Multiport Switch : MultiPortSwitch  DataPortOrder=Zero-based contiguous  Inputs=2  zeroidx=on
  Signal Override Switch 0 = Use Model 1 = Use Constant : Constant  Value=0
  Out1 : Outport
  wires:
  Constant/1 -> Multiport Switch/3
  Multiport Switch/1 -> Out1/1
  In1/1 -> Multiport Switch/2
  Signal Override Switch 0 = Use Model 1 = Use Constant/1 -> Multiport Switch/1

== system P2_SIL_Model_Diag/Fault Trigger Unit/Component Diagnostics setting/Override  MCUOverTemp ==
  note: This subsystem is used to override the model value of a signal to a constant value
  note: Override Switch Subsystem
  In1 : Inport
  Constant : Constant  Value=0
  Multiport Switch : MultiPortSwitch  DataPortOrder=Zero-based contiguous  Inputs=2  zeroidx=on
  Signal Override Switch 0 = Use Model 1 = Use Constant : Constant  Value=0
  Out1 : Outport
  wires:
  Signal Override Switch 0 = Use Model 1 = Use Constant/1 -> Multiport Switch/1
  In1/1 -> Multiport Switch/2
  Multiport Switch/1 -> Out1/1
  Constant/1 -> Multiport Switch/3

== system P2_SIL_Model_Diag/Fault Trigger Unit/Component Diagnostics setting/Override  MotDirMismatch ==
  note: Override Switch Subsystem
  note: This subsystem is used to override the model value of a signal to a constant value
  In1 : Inport
  Constant : Constant  Value=0
  Multiport Switch : MultiPortSwitch  DataPortOrder=Zero-based contiguous  Inputs=2  zeroidx=on
  Signal Override Switch 0 = Use Model 1 = Use Constant : Constant  Value=0
  Out1 : Outport
  wires:
  Constant/1 -> Multiport Switch/3
  Multiport Switch/1 -> Out1/1
  In1/1 -> Multiport Switch/2
  Signal Override Switch 0 = Use Model 1 = Use Constant/1 -> Multiport Switch/1

== system P2_SIL_Model_Diag/Fault Trigger Unit/Component Diagnostics setting/Override  MotOverTemp ==
  note: Override Switch Subsystem
  note: This subsystem is used to override the model value of a signal to a constant value
  In1 : Inport
  Constant : Constant  Value=0
  Multiport Switch : MultiPortSwitch  DataPortOrder=Zero-based contiguous  Inputs=2  zeroidx=on
  Signal Override Switch 0 = Use Model 1 = Use Constant : Constant  Value=0
  Out1 : Outport
  wires:
  Constant/1 -> Multiport Switch/3
  Multiport Switch/1 -> Out1/1
  In1/1 -> Multiport Switch/2
  Signal Override Switch 0 = Use Model 1 = Use Constant/1 -> Multiport Switch/1

== system P2_SIL_Model_Diag/Fault Trigger Unit/Component Diagnostics setting/Override  MotTrqMismatch ==
  note: This subsystem is used to override the model value of a signal to a constant value
  note: Override Switch Subsystem
  In1 : Inport
  Constant : Constant  Value=0
  Multiport Switch : MultiPortSwitch  DataPortOrder=Zero-based contiguous  Inputs=2  zeroidx=on
  Signal Override Switch 0 = Use Model 1 = Use Constant : Constant  Value=0
  Out1 : Outport
  wires:
  Signal Override Switch 0 = Use Model 1 = Use Constant/1 -> Multiport Switch/1
  In1/1 -> Multiport Switch/2
  Multiport Switch/1 -> Out1/1
  Constant/1 -> Multiport Switch/3

== system P2_SIL_Model_Diag/Fault Trigger Unit/Driver Interface Diagnostics setting/Override  APP1_OOR ==
  note: Override Switch Subsystem
  note: This subsystem is used to override the model value of a signal to a constant value
  In1 : Inport
  Constant : Constant  Value=0
  Multiport Switch : MultiPortSwitch  DataPortOrder=Zero-based contiguous  Inputs=2  zeroidx=on
  Signal Override Switch 0 = Use Model 1 = Use Constant : Constant  Value=0
  Out1 : Outport
  wires:
  Constant/1 -> Multiport Switch/3
  Multiport Switch/1 -> Out1/1
  In1/1 -> Multiport Switch/2
  Signal Override Switch 0 = Use Model 1 = Use Constant/1 -> Multiport Switch/1

== system P2_SIL_Model_Diag/Fault Trigger Unit/Driver Interface Diagnostics setting/Override  APP2_OOR ==
  note: This subsystem is used to override the model value of a signal to a constant value
  note: Override Switch Subsystem
  In1 : Inport
  Constant : Constant  Value=0
  Multiport Switch : MultiPortSwitch  DataPortOrder=Zero-based contiguous  Inputs=2  zeroidx=on
  Signal Override Switch 0 = Use Model 1 = Use Constant : Constant  Value=0
  Out1 : Outport
  wires:
  Signal Override Switch 0 = Use Model 1 = Use Constant/1 -> Multiport Switch/1
  In1/1 -> Multiport Switch/2
  Multiport Switch/1 -> Out1/1
  Constant/1 -> Multiport Switch/3

== system P2_SIL_Model_Diag/Fault Trigger Unit/Driver Interface Diagnostics setting/Override  APP_Mismatch ==
  note: Signal Override Switch
      | 0 = Use Model
      | 1 = Use Constant
  note: Override Switch Subsystem
  note: This subsystem is used to override the model value of a signal to a constant value
  In1 : Inport
  APP_Mismatch_Override : Constant  Value=0
  Constant : Constant  Value=0
  Multiport Switch : MultiPortSwitch  DataPortOrder=Zero-based contiguous  Inputs=2  zeroidx=on
  Out1 : Outport
  wires:
  Constant/1 -> Multiport Switch/3
  Multiport Switch/1 -> Out1/1
  In1/1 -> Multiport Switch/2
  APP_Mismatch_Override/1 -> Multiport Switch/1

== system P2_SIL_Model_Diag/Fault Trigger Unit/Driver Interface Diagnostics setting/Override  BPP_Flt ==
  note: This subsystem is used to override the model value of a signal to a constant value
  note: Override Switch Subsystem
  In1 : Inport
  Constant : Constant  Value=0
  Multiport Switch : MultiPortSwitch  DataPortOrder=Zero-based contiguous  Inputs=2  zeroidx=on
  Signal Override Switch 0 = Use Model 1 = Use Constant : Constant  Value=0
  Out1 : Outport
  wires:
  Signal Override Switch 0 = Use Model 1 = Use Constant/1 -> Multiport Switch/1
  In1/1 -> Multiport Switch/2
  Multiport Switch/1 -> Out1/1
  Constant/1 -> Multiport Switch/3

== system P2_SIL_Model_Diag/Fault Trigger Unit/Driver Interface Diagnostics setting/Override  KeyPos_Flt ==
  note: Override Switch Subsystem
  note: This subsystem is used to override the model value of a signal to a constant value
  In1 : Inport
  Constant : Constant  Value=0
  Multiport Switch : MultiPortSwitch  DataPortOrder=Zero-based contiguous  Inputs=2  zeroidx=on
  Signal Override Switch 0 = Use Model 1 = Use Constant : Constant  Value=0
  Out1 : Outport
  wires:
  Constant/1 -> Multiport Switch/3
  Multiport Switch/1 -> Out1/1
  In1/1 -> Multiport Switch/2
  Signal Override Switch 0 = Use Model 1 = Use Constant/1 -> Multiport Switch/1

== system P2_SIL_Model_Diag/Fault Trigger Unit/Driver Interface Diagnostics setting/Override  PRNDL_Flt ==
  note: This subsystem is used to override the model value of a signal to a constant value
  note: Override Switch Subsystem
  In1 : Inport
  Constant : Constant  Value=0
  Multiport Switch : MultiPortSwitch  DataPortOrder=Zero-based contiguous  Inputs=2  zeroidx=on
  Signal Override Switch 0 = Use Model 1 = Use Constant : Constant  Value=0
  Out1 : Outport
  wires:
  Signal Override Switch 0 = Use Model 1 = Use Constant/1 -> Multiport Switch/1
  In1/1 -> Multiport Switch/2
  Multiport Switch/1 -> Out1/1
  Constant/1 -> Multiport Switch/3

== system P2_SIL_Model_Diag/Plant Actuators/Analog/APP_Fault_Insertion ==
  AccPos : Inport
  Constant : Constant  Value=0
  Constant1 : Constant  Value=cal.APP.Mismatch_Value+0.1
  Constant2 : Constant  Value=0
  Constant3 : Constant  Value=cal.APP2.IN_Max_SC_Prcnt+1
  Constant4 : Constant  Value=0
  Constant5 : Constant  Value=cal.APP1.IN_Max_SC_Prcnt+1
  Sum1 : Sum  Inputs=+++
  Sum2 : Sum
  Switch : Switch  Threshold=1
  Switch1 : Switch  Threshold=1
  Switch2 : Switch  Threshold=1
  APP1 : Outport
  APP2 : Outport  Port=2
  wires:
  Constant5/1 -> Switch2/1
  [APP1_OOR_ON] -> Switch2/2
  Constant4/1 -> Switch2/3
  Switch2/1 -> Sum2/1
  Sum2/1 -> APP1/1
  [Mismatch_APP_ON] -> Switch/2
  Switch/1 -> Sum1/2
  Constant/1 -> Switch/3
  Constant2/1 -> Switch1/3
  Constant3/1 -> Switch1/1
  [APP2_OOR_ON] -> Switch1/2
  Switch1/1 -> Sum1/3
  Constant1/1 -> Switch/1
  AccPos/1 -> Sum2/2, Sum1/1
  Sum1/1 -> APP2/1

== system P2_SIL_Model_Diag/Plant Actuators/Analog/APP_to_APP1_Recast ==
  APP1_IN : Inport
  APP1_Recast_Max : Constant  Value=cal.APP1.IN_Max
  APP1_Recast_Min : Constant  Value=cal.APP1.IN_Min
  Gain1 : Gain  Gain=1/100
  Product1 : Product  RndMeth=Zero
  Sum1 : Sum  Inputs=|+-
  Sum2 : Sum  Inputs=|++
  APP1Recast : Outport
  wires:
  APP1_IN/1 -> Gain1/1
  Sum2/1 -> APP1Recast/1
  APP1_Recast_Max/1 -> Sum1/1
  APP1_Recast_Min/1 -> Sum2/2, Sum1/2
  Sum1/1 -> Product1/2
  Gain1/1 -> Product1/1
  Product1/1 -> Sum2/1

== system P2_SIL_Model_Diag/Plant Actuators/Analog/APP_to_APP2_Recast ==
  APP2_IN : Inport
  APP2_Recast_Max : Constant  Value=cal.APP2.IN_Max
  APP2_Recast_Min : Constant  Value=cal.APP2.IN_Min
  Gain1 : Gain  Gain=1/100
  Product1 : Product  RndMeth=Zero
  Sum1 : Sum  Inputs=|+-
  Sum2 : Sum  Inputs=|++
  APP2Recast : Outport
  wires:
  APP2_IN/1 -> Gain1/1
  Sum2/1 -> APP2Recast/1
  APP2_Recast_Max/1 -> Sum1/1
  APP2_Recast_Min/1 -> Sum2/2, Sum1/2
  Sum1/1 -> Product1/2
  Gain1/1 -> Product1/1
  Product1/1 -> Sum2/1

== system P2_SIL_Model_Diag/Plant Actuators/CAN/EBCAN ==
  In1 : Inport
  BMS_Antrieb : Subsystem
  Bus Creator : BusCreator  Inputs=2
  ECM : Subsystem
  Out1 : Outport
  wires:
  Bus Creator/1 -> Out1/1  "EBCAN"
  BMS_Antrieb/1(Out1) -> Bus Creator/2
  ECM/1(Out1) -> Bus Creator/1
  In1/1 -> ECM/1(In1), BMS_Antrieb/1(In1)

== system P2_SIL_Model_Diag/Plant Actuators/CAN/HV_CAN ==
  In1 : Inport
  APM : Subsystem  Commented=on
  BMS_Hybrid : Subsystem
  Bus Creator : BusCreator  Inputs=4
  MCU : Subsystem
  OBC : Subsystem
  Out1 : Outport
  wires:
  In1/1 -> BMS_Hybrid/1(In1), MCU/1(In1), OBC/1(In1), APM/1(In1)
  Bus Creator/1 -> Out1/1  "HV_CAN"
  OBC/1(Out1) -> Bus Creator/3
  MCU/1(Out1) -> Bus Creator/2
  BMS_Hybrid/1(Out1) -> Bus Creator/1

== system P2_SIL_Model_Diag/Plant Actuators/CAN/VEH_CAN ==
  In1 : Inport
  BCM : Subsystem
  Bus Creator : BusCreator  Inputs=4
  Bus Selector : BusSelector  OutputSignals=TCM_CAN,BCM_CAN
  EBCM : Subsystem
  Ground : Ground
  Ground1 : Ground
  ICCM : Subsystem
  TCM : Subsystem
  Out1 : Outport
  wires:
  Ground1/1 -> ICCM/1(In1)
  Ground/1 -> EBCM/1(In1)
  BCM/1(Out1) -> Bus Creator/2
  EBCM/1(Out1) -> Bus Creator/3
  Bus Selector/2 -> BCM/1(In1)  "<BCM_CAN>"
  Bus Selector/1 -> TCM/1(In1)  "<TCM_CAN>"
  In1/1 -> Bus Selector/1
  Bus Creator/1 -> Out1/1  "VEH_CAN"
  ICCM/1(Out1) -> Bus Creator/4
  TCM/1(Out1) -> Bus Creator/1

== system P2_SIL_Model_Diag/Plant Sensors/CAN/EBCAN ==
  In1 : Inport
  BMS_Antrieb : Subsystem
  Bus Creator : BusCreator  Inputs=2
  ECM : Subsystem
  Out1 : Outport
  wires:
  Bus Creator/1 -> Out1/1
  BMS_Antrieb/1(Out1) -> Bus Creator/2
  ECM/1(Out1) -> Bus Creator/1
  In1/1 -> ECM/1(In1), BMS_Antrieb/1(In1)

== system P2_SIL_Model_Diag/Plant Sensors/CAN/HV_CAN ==
  In1 : Inport
  APM : Subsystem  Commented=on
  BMS_Hybrid : Subsystem
  Bus Creator : BusCreator  Inputs=4
  MCU : Subsystem
  OBC : Subsystem
  Out1 : Outport
  wires:
  APM/1(Out1) -> Bus Creator/4
  In1/1 -> BMS_Hybrid/1(In1), MCU/1(In1), OBC/1(In1), APM/1(In1)
  Bus Creator/1 -> Out1/1
  OBC/1(Out1) -> Bus Creator/3
  MCU/1(Out1) -> Bus Creator/2
  BMS_Hybrid/1(Out1) -> Bus Creator/1

== system P2_SIL_Model_Diag/Plant Sensors/CAN/VEH_CAN ==
  In1 : Inport
  BCM : Subsystem
  Bus Creator : BusCreator  Inputs=4
  EBCM : Subsystem
  ICCM : Subsystem
  TCM : Subsystem
  Out1 : Outport
  wires:
  In1/1 -> ICCM/1(In1), BCM/1(In1), EBCM/1(In1), TCM/1(In1)
  Bus Creator/1 -> Out1/1
  ICCM/1(Out1) -> Bus Creator/4  "to_ICCM"
  BCM/1(Out1) -> Bus Creator/3  "to_BCM"
  EBCM/1(Out1) -> Bus Creator/2  "to_EBCM"
  TCM/1(Out1) -> Bus Creator/1  "to_TCM"

== system P2_SIL_Model_Diag/Sensors/Analog/APP Manipulation ==
  note: $Author: eo1000 $
      | $Rev: 296 $
      | $Date: 2013-11-14 10:37:07 -0500 (Thu, 14 Nov 2013) $
  APP1_IN : Inport
  APP2_IN : Inport  Port=2
  APP1_Conversion : Subsystem
  APP2_Conversion : Subsystem
  Bus Creator1 : BusCreator  Inputs=4
  APP : Outport
  wires:
  APP2_IN/1 -> APP2_Conversion/1(APP2_IN)
  APP2_Conversion/1(APP2) -> Bus Creator1/4  "APP_Norm_Pos2"
  APP1_Conversion/1(APP1) -> Bus Creator1/3  "APP_Norm_Pos1"
  APP1_IN/1 -> APP1_Conversion/1(APP1_IN)
  Bus Creator1/1 -> APP/1
  APP1_Conversion/2(OOR) -> Bus Creator1/1  "APP1_OOR"
  APP2_Conversion/2(OOR) -> Bus Creator1/2  "APP2_OOR"

== system P2_SIL_Model_Diag/Sensors/CAN/EBCAN ==
  In1 : Inport
  BMS_Antrieb : Subsystem
  Bus Creator : BusCreator  Inputs=3
  Bus Selector : BusSelector  OutputSignals=EBCAN.ECM_CAN,EBCAN.BMS_Hybrid
  CCM : Subsystem
  Constant : Constant
  ECM : Subsystem
  Out1 : Outport
  wires:
  ECM/1(Out1) -> Bus Creator/1  "from_ECM"
  BMS_Antrieb/1(Out1) -> Bus Creator/2  "from_BMSAntrieb"
  Bus Creator/1 -> Out1/1
  CCM/1(Out1) -> Bus Creator/3  "from_CCM"
  In1/1 -> Bus Selector/1
  Bus Selector/1 -> ECM/1(In1)  "<ECM_CAN>"
  Bus Selector/2 -> BMS_Antrieb/1(In1)  "<BMS_Hybrid>"
  Constant/1 -> CCM/1(In1)

== system P2_SIL_Model_Diag/Sensors/CAN/HV_CAN ==
  In1 : Inport
  APM : Subsystem  Commented=on
  BMS_Hybrid : Subsystem
  Bus Creator : BusCreator  Inputs=4
  Bus Selector : BusSelector  OutputSignals=HV_CAN.MCU_CAN,HV_CAN.BMS_Plugin,HV_CAN.OBC_CAN
  MCU : Subsystem
  OBC : Subsystem
  Out1 : Outport
  wires:
  MCU/1(Out1) -> Bus Creator/1  "from_MCU"
  BMS_Hybrid/1(Out1) -> Bus Creator/2  "from_BMSHybrid"
  OBC/1(Out1) -> Bus Creator/3  "from_OBC"
  Bus Creator/1 -> Out1/1
  APM/1(Out1) -> Bus Creator/4  "from_APM"
  In1/1 -> Bus Selector/1
  Bus Selector/1 -> MCU/1(In1)  "<MCU_CAN>"
  Bus Selector/2 -> BMS_Hybrid/1(In1)  "<BMS_Plugin>"
  Bus Selector/3 -> OBC/1(In1)  "<OBC_CAN>"

== system P2_SIL_Model_Diag/Sensors/CAN/VEH_CAN ==
  In1 : Inport
  BCM : Subsystem
  Bus Creator : BusCreator  Inputs=4
  Bus Selector : BusSelector  OutputSignals=VEH_CAN.TCM_CAN,VEH_CAN.BCM_CAN,VEH_CAN.signal3,VEH_CAN.signal4
  EBCM : Subsystem
  ICCM : Subsystem
  TCM : Subsystem
  Out1 : Outport
  wires:
  In1/1 -> Bus Selector/1
  TCM/1(Out1) -> Bus Creator/1  "from_TCM"
  BCM/1(Out1) -> Bus Creator/2  "from_BCM"
  ICCM/1(Out1) -> Bus Creator/3  "from_ICCM"
  EBCM/1(Out1) -> Bus Creator/4  "from_EBCM"
  Bus Creator/1 -> Out1/1
  Bus Selector/1 -> TCM/1(In1)  "<TCM_CAN>"
  Bus Selector/2 -> BCM/1(In1)  "<BCM_CAN>"
  Bus Selector/3 -> ICCM/1(In1)  "<signal3>"
  Bus Selector/4 -> EBCM/1(In1)  "<signal4>"

== system P2_SIL_Model_Diag/Actuators/CAN/EBCAN/BMS_Antrieb ==
  In1 : Inport
  Bus Selector : BusSelector  OutputSignals=BMS_CAN.ISO_Funktionaler_Req_All
  Out1 : Outport
  wires:
  In1/1 -> Bus Selector/1
  Bus Selector/1 -> Out1/1  "<ISO_Funktionaler_Req_All>"

== system P2_SIL_Model_Diag/Actuators/CAN/EBCAN/ECM ==
  In1 : Inport
  Bus Creator : BusCreator  Inputs=4
  Bus Selector : BusSelector  OutputSignals=Controls.EngAppReq,Controls.EngOnReq,Controls.EngTrqCmd,Controls.ShftLvrPos
  Out1 : Outport
  wires:
  In1/1 -> Bus Selector/1
  Bus Selector/1 -> Bus Creator/1  "<EngAppReq>"
  Bus Selector/2 -> Bus Creator/2  "<EngOnReq>"
  Bus Selector/3 -> Bus Creator/3  "<EngTrqCmd>"
  Bus Creator/1 -> Out1/1  "ECM_CAN"
  Bus Selector/4 -> Bus Creator/4  "<ShftLvrPos>"

== system P2_SIL_Model_Diag/Actuators/CAN/HV_CAN/APM ==
  In1 : Inport
  Bus Selector : BusSelector  OutputSignals=APM_CAN
  Out1 : Outport
  wires:
  In1/1 -> Bus Selector/1
  Bus Selector/1 -> Out1/1  "<APM_CAN>"

== system P2_SIL_Model_Diag/Actuators/CAN/HV_CAN/BMS_Hybrid ==
  In1 : Inport
  Bus Creator : BusCreator  Inputs=2
  Bus Selector : BusSelector  OutputSignals=BMS_CAN.MSG_HYB_01,Controls.MO_BMS_Sollmodus
  Out1 : Outport
  wires:
  In1/1 -> Bus Selector/1
  Bus Selector/1 -> Bus Creator/1  "<MSG_HYB_01>"
  Bus Selector/2 -> Bus Creator/2  "<MO_BMS_Sollmodus>"
  Bus Creator/1 -> Out1/1
